simulink library "PFB"  (R2018a)
settings: Solver=VariableStepAuto  StartTime=0.0  StopTime=10.0  RelTol=1e-3
libraries: xbsIndex_r4 x1
settings Model: Creator=mybur  LastModifiedBy=mybur
settings DataIOCC: ReturnWorkspaceOutputs=on
settings SFSimCC: SimUseLocalCustomCode=on
settings RTWCC: RTWUseLocalCustomCode=on

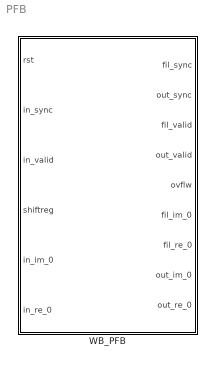
== system PFB ==
  WB_PFB : Subsystem  mask{use_reorder=on, use_fft_shift=on, use_separate=on, wb_factor=1, nof_points=1024, win="hanning", fwidth=1.0, nof_taps=1, nof_wb_streams=1, nof_chan=1, backoff_w=0, xtra_dat_sigs=off, big_endian_wb_in=on, use_prefilter=on, dont_flip_channels=on, fft_in_dat_w=10, fil_in_dat_w=10, fft_out_dat_w=10, fil_out_dat_w=10, out_gain_w=0, fft_stage_dat_w=10, fil_coef_dat_w=10, fft_guard_enable=on, fft_guard_w=2, fft_ovflw_behav="WRAP", fft_use_round="ROUND", use_variant="4DSP", use_dsp="YES", fft_ram_primitive="block", fil_ram_primitive="block", fifo_primitive="block", vendor_technology=Xilinx}
      mask prompts: use_reorder "Bit reverse output"; use_fft_shift "Reorder frequencies"; use_separate "Separate re/im outputs"; wb_factor "Wideband factor"; nof_points "Number of points"; win "Window function"; nof_taps "Number of taps"; nof_wb_streams "Number of wideband streams"; nof_chan "Number of channels"; backoff_w "Filter backoff width"; xtra_dat_sigs "Extra control signals"; big_endian_wb_in "Big endian input data"; use_prefilter "Enable prefilter"; dont_flip_channels "Don't flip channels"; fft_in_dat_w "FFT Input data widths"; fil_in_dat_w "Prefilter input data width"; fft_out_dat_w "FFT output data width"; fil_out_dat_w "Prefilter output data width"; out_gain_w "Output gain width"; fft_stage_dat_w "FFT stage data width"; fil_coef_dat_w "Prefilter coefficient data width"; fft_guard_enable "Guard FFT input data"; fft_guard_w "FFT guard data width"; fft_ovflw_behav "FFT overflow behaviour"; fft_use_round "FFT rounding behaviour"; use_variant "Use 3DSP or 4DSP multipliers"; use_dsp "Use DSP48 for cmults"; fft_ram_primitive "FFT Ram Primitive"; fil_ram_primitive "Prefilter Ram Primitive"; fifo_primitive "Fifo Primitive"; vendor_technology "Vendor technology"
      mask init:
      | Simulink.Block.eval([gcb, '/wb_pfb']);
      |  
      | wb_pfb_subsys2bb_knit();
      mask TypeOptions win: "hanning" | "hamming" | "blackman"
      mask TypeOptions fft_ovflw_behav: "SATURATE" | "WRAP"
      mask TypeOptions fft_use_round: "TRUNCATE" | "ROUND"
      mask TypeOptions use_variant: "4DSP" | "3DSP"
      mask TypeOptions use_dsp: "YES" | "NO"
      mask TypeOptions fft_ram_primitive: "block" | "distributed" | "ultra" | "auto"
      mask TypeOptions fil_ram_primitive: "block" | "distributed" | "ultra" | "auto"
      mask TypeOptions fifo_primitive: "block" | "distributed" | "ultra" | "auto"
      mask TypeOptions vendor_technology: Xilinx | UniBoard
      mask DialogControl pfb_params Prompt: PFB Parameters
      mask DialogControl data_params Prompt: Data Parameters
      mask DialogControl fpga_params Prompt: FPGA Parameters

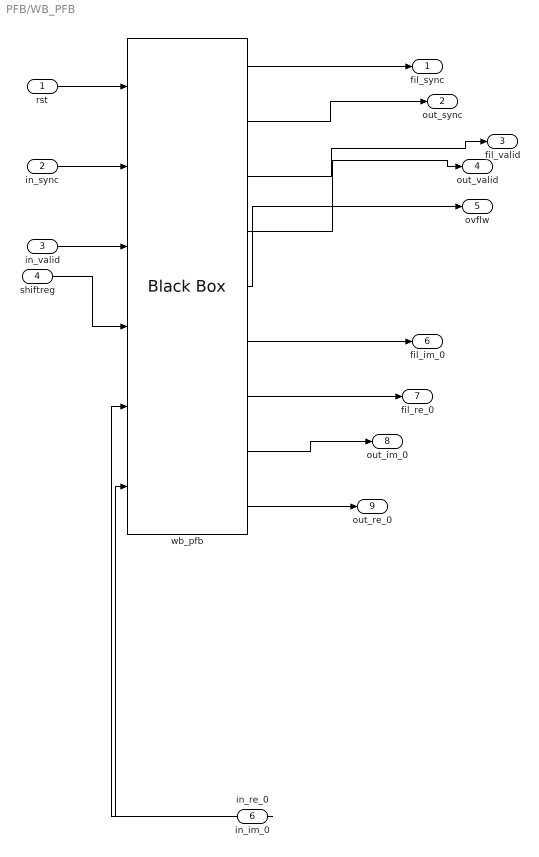
== system PFB/WB_PFB ==
  rst : Inport
  in_sync : Inport  Port=2
  in_valid : Inport  Port=3
  shiftreg : Inport  Port=4
  in_im_0 : Inport  Port=5
  in_re_0 : Inport  Port=6
  wb_pfb : xbsIndex_r4/Black Box  init_code=wbpfb_unit_top_config  sim_method=ISE Simulator  verbose=off  block_type=blackbox2
  fil_sync : Outport
  out_sync : Outport  Port=2
  fil_valid : Outport  Port=3
  out_valid : Outport  Port=4
  ovflw : Outport  Port=5
  fil_im_0 : Outport  Port=6
  fil_re_0 : Outport  Port=7
  out_im_0 : Outport  Port=8
  out_re_0 : Outport  Port=9
  wires:
  wb_pfb/9 -> out_re_0/1
  wb_pfb/8 -> out_im_0/1
  wb_pfb/7 -> fil_re_0/1
  wb_pfb/6 -> fil_im_0/1
  in_re_0/1 -> wb_pfb/6
  in_im_0/1 -> wb_pfb/5
  wb_pfb/5 -> ovflw/1
  wb_pfb/4 -> out_valid/1
  wb_pfb/3 -> fil_valid/1
  wb_pfb/2 -> out_sync/1
  wb_pfb/1 -> fil_sync/1
  shiftreg/1 -> wb_pfb/4
  in_valid/1 -> wb_pfb/3
  in_sync/1 -> wb_pfb/2
  rst/1 -> wb_pfb/1
